simulink model "mulaw2"  (Simulink 10.0)
settings: Solver=ode45  StartTime=0.0  StopTime=inf  RelTol=1e-3  EnableMultiTasking=on
libraries: commsrccod2 x2, dspsrcs4 x1, dspsnks4 x1
settings Model: Creator=Kerry Schutz  LastModifiedBy=bhisma
settings DataIOCC: LimitDataPoints=on  SignalLoggingSaveFormat=ModelDataLogs
settings OptimizationCC: ExpressionDepthLimit=2147483647  InitFltsAndDblsToZero=on
settings DebuggingCC: SolverPrmCheckMsg=warning  FcnCallInpInsideContextMsg=warning  StateNameClashWarn=warning
settings SFSimCC: SimUseLocalCustomCode=on  CustomCodeUndefinedFunction=FilterOut
settings RTWCC: RTWUseLocalCustomCode=on

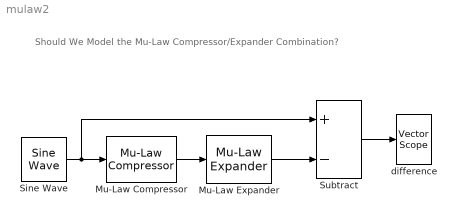
== system mulaw2 ==
  note: Should We Model the Mu-Law Compressor/Expander Combination?
  Mu-Law Compressor : commsrccod2/Mu-Law Compressor  SystemSampleTime=-1  mu=255  V=1
      settings: SourceProductName=Communications Toolbox  SourceProductBaseCode=CM
  Mu-Law Expander : commsrccod2/Mu-Law Expander  SystemSampleTime=-1  mu=255  V=1
      settings: SourceProductName=Communications Toolbox  SourceProductBaseCode=CM
  Sine Wave : dspsrcs4/Sine Wave  Amplitude=1  Frequency=200  Phase=0  SampleMode=Discrete  OutComplex=Real  CompMethod=Trigonometric fcn  TableSize=Speed  SampleTime=1/8000  SamplesPerFrame=80  dataType=double  wordLen=16  udDataType=sfix(16)  fracBitsMode=Best precision  numFracBits=15  ResetState=Restart at time zero
  Subtract : Sum  Inputs=+-
  difference : dspsnks4/Vector Scope  ScopeProperties=on  Domain=Time  HorizSpan=1  DisplayProperties=off  AxisGrid=on  Memory=off  FrameNumber=on  AxisLegend=off  AxisZoom=off  OpenScopeAtSimStart=on  OpenScopeImmediately=off  FigPos=[231 308 359 191]  AxisProperties=off  XUnits=Hertz  XRange=[0...Fs/2]  InheritXIncr=on  XIncr=1  XLabel=Time  XLimit=Auto  XMin=0  XMax=1  XStart=0  YUnits=dB  YLabel=Amplitude  LineProperties=off
      settings: SourceProductName=DSP System Toolbox  SourceProductBaseCode=DS  YMin=-1.32116539930394e-015  YMax=8.82072193064687e-016
  wires:
  Sine Wave/1 -> Mu-Law Compressor/1, Subtract/1
  Mu-Law Compressor/1 -> Mu-Law Expander/1
  Mu-Law Expander/1 -> Subtract/2
  Subtract/1 -> difference/1
